simulink model "CRCL"  (R2020b)
settings: Solver=FixedStepDiscrete  StartTime=0.0  StopTime=inf  FixedStep=0.01  RelTol=1e-3  EnableMultiTasking=on
values from neighbouring files (symbols this model uses):
  calibrationDelayTime_s = 2.0    [CRCL_Dictionary.sldd]
  collisionAngleThreshold_deg = 40.0    [CRCL_Dictionary.sldd]
  collisionVarianceThreshold_g2 = 8.0    [CRCL_Dictionary.sldd]
  cpMaxAbortTime_s = 30.0    [CRCL_Dictionary.sldd]
  cpMaxTipOverAngle_deg = 35.0    [CRCL_Dictionary.sldd]
  cpMinEstDistance_m = 50.0    [CRCL_Dictionary.sldd]
  cpMinEstDistanceGnssBased_m = 200.0    [CRCL_Dictionary.sldd]
  cpMinRiddenTime_s = 15.0    [CRCL_Dictionary.sldd]
  cpMinSpeedRiding_kmh = 10.0    [CRCL_Dictionary.sldd]
  cpNumCrankRevolutionThreshold = 5.0    [CRCL_Dictionary.sldd]
  cpSpeedCond2PositiveSpeedChangeTime_s = 5.0    [CRCL_Dictionary.sldd]
  cpSpeedDerivativeThreshold_kmhs = 0.005    [CRCL_Dictionary.sldd]
  cpTimeOutSpeedCond2_s = 15.0    [CRCL_Dictionary.sldd]
  groundHitEnergyThresholdStanding_g2s2 = 0.02    [CRCL_Dictionary.sldd]
  groundHitTipOverAngleThreshold_deg = 40.0    [CRCL_Dictionary.sldd]
  longAccCompForEulerEstFlag = 0.0    [CRCL_Dictionary.sldd]
  minEnergyStrongHit_g2s2 = 0.1    [CRCL_Dictionary.sldd]
  noMotionAccVarianceThresholdSD_g2 = 0.001    [CRCL_Dictionary.sldd]
  ride1minSpeedSlow_kmh = 4.0    [CRCL_Dictionary.sldd]
  ride2minSpeed_kmh = 8.0    [CRCL_Dictionary.sldd]
  rroMaxSpeed_kmh = 5.0    [CRCL_Dictionary.sldd]
  rroMinGyrX_degs = 20.0    [CRCL_Dictionary.sldd]
  rroMonotonyThreshold_degs = -1.0    [CRCL_Dictionary.sldd]
  rroRollIntegrationAngleThreshold_degs = 20.0    [CRCL_Dictionary.sldd]
  rroUniContinuityThreshold_degs = 15.0    [CRCL_Dictionary.sldd]
  scaleFactorVarianceStrongHit = 2.0    [CRCL_Dictionary.sldd]
  sdoMaxAccVarFreeFall_g2 = 0.06    [CRCL_Dictionary.sldd]
  sdoMaxTipOverAngle_deg = 20.0    [CRCL_Dictionary.sldd]
  sdoMinAccVar_g2 = 8.0    [CRCL_Dictionary.sldd]
  sdoMinGyrXYNorm_degs = 720.0    [CRCL_Dictionary.sldd]
  sdoMinGyrXYNormFreeFall_degs = 100.0    [CRCL_Dictionary.sldd]
  sdoMinOrientationChange_deg = 120.0    [CRCL_Dictionary.sldd]
  sdoScaleFactorOrientationChange = 3.0    [CRCL_Dictionary.sldd]
  stepTime_s = 0.01    [CRCL_Dictionary.sldd]
  strongHitSafetyFactor = 2.5    [CRCL_Dictionary.sldd]
  tipOverAccZFiltTreshold_g = 0.7    [CRCL_Dictionary.sldd]
  tipOverAngleThreshold_deg = 50.0    [CRCL_Dictionary.sldd]
  tipOverMinAccZFiltNoseOver_g = 0.3    [CRCL_Dictionary.sldd]
  tipOverRollPitchRelationNoseOver = 1.5    [CRCL_Dictionary.sldd]
undefined symbols (not defined in the file or in its folder): magnitude
libraries: simulink x17
(part 5 of 8)

== stateflow chart CRCL/BikeCrashFusionProduct ==
  state CrashFusionAndDetection_SchneeV2_softHit2 [parallel] [commented out]
    state Init [commented out]
      en:
      CF_fire = int16(0);
      CF_checkTipOverTimeDelay = single(2);
      CF_possibleTo = single(0);
      HD_GroundHitFireIntern = int16(0);
      HD_CollisionHitFireIntern = int16(0);
    state RidingNotCalibratedTipOver [commented out]
      en:
      CF_fire = int16(1);
      CF_scenario = int16(70);
    state RidingNotCalibrated [commented out]
      en:
    state NoCrash [commented out]
      en:
      CF_scenario = int16(0);
      HD_CollisionHitFireIntern = int16(0);
      HD_GroundHitFireIntern = int16(0);
      du:
      CF_possibleTo = single(0);
    state waitUntilBikeIsUprightAgain [commented out]
    state wait2 [commented out]
      en:
      if CF_possibleTo == 0
      RD_fireIntern = RD_fire;
      end
      if HD_CollisionHitFire ==  1
      HD_CollisionHitFireIntern = int16(1);
      end
      CF_possibleTo = single(1);
    state HitDetected [commented out]
      %wait for possible Ground Hit and TipOver
      en:
      du:
      if HD_CollisionHitFire ==  3
      HD_CollisionHitFireIntern = int16(3);
      end
      if HD_GroundHitFire == 1
      HD_GroundHitFireIntern = int16(1);
      end
    state wait1 [commented out]
      en:
      if CF_possibleTo == 0
      RD_fireIntern = RD_fire;
      end
      if HD_CollisionHitFire ==  3
      HD_CollisionHitFireIntern = int16(3);
      elseif HD_CollisionHitFire ==  2
      HD_CollisionHitFireIntern = int16(2);
      elseif HD_CollisionHitFire ==  1
      HD_CollisionHitFireIntern = int16(1);
      end
      du:
      if HD_CollisionHitFire ==  2 && HD_CollisionHitFireIntern < 2
      HD_CollisionHitFireIntern = int16(2);
      end
      if HD_CollisionHitFire == 3 && HD_CollisionHitFireIntern < 3
      HD_CollisionHitFireIntern = int16(3);
      end
    state wait [commented out]
      du:
      if HD_GroundHitFire == 1
      HD_GroundHitFireIntern = int16(1);
      end
      ex:
      if HD_GroundHitFire == 1
      HD_GroundHitFireIntern = int16(1);
      end
      if HD_CollisionHitFire ==  3
      HD_CollisionHitFireIntern = int16(3);
      elseif HD_CollisionHitFire ==  2
      HD_CollisionHitFireIntern = int16(2);
      elseif HD_CollisionHitFire ==  1
      HD_CollisionHitFireIntern = int16(1);
      end
    note: ______________________________________________________________________________________________________________________________________________________________________________________________v Ride Feature Layer v
    note: ______________________________________________________________________________________________________________________________________________________________________________________________v CollisionHit Feature Layer v
    note: ______________________________________________________________________________________________________________________________________________________________________________________________v GroundHit Feature Layer v
    note: ____________________________________________________________________________________________________________________________________________________________________________________________________________v TipOver Feature Layer v
    note: ____________________________________________________________________________________________________________________________________________________________________________________________________________v StrongHit Feature Layer v
    note: _________________________________________________________________________________________________________________________________________________________________________________________________________________v Classifcation Layer v
    state Crash [commented out]
      en:
      if ~(CF_scenario == 70)
      CF_fire = int16(1);
      end
    (default) -> CrashFusionAndDetection_SchneeV2_softHit2.Init [commented out]
    CrashFusionAndDetection_SchneeV2_softHit2.RidingNotCalibratedTipOver -> CrashFusionAndDetection_SchneeV2_softHit2.Init [commented out] : [after(5,sec) && TO_fire == 0]
        | {
        | CF_fire = int16(0);
        | CF_scenario = int16(0);
        | }
    CrashFusionAndDetection_SchneeV2_softHit2.RidingNotCalibrated -> CrashFusionAndDetection_SchneeV2_softHit2.Init [commented out] : [RD_fire < 2]
    CrashFusionAndDetection_SchneeV2_softHit2.RidingNotCalibrated -> CrashFusionAndDetection_SchneeV2_softHit2.RidingNotCalibratedTipOver [commented out] : [TO_fire == 3]
    CrashFusionAndDetection_SchneeV2_softHit2.Init -> CrashFusionAndDetection_SchneeV2_softHit2.RidingNotCalibrated [commented out] : [CF_systemConfig == 2 && RD_fire >= 2 && TO_fire ~= 3]
    CrashFusionAndDetection_SchneeV2_softHit2.RidingNotCalibrated -> CrashFusionAndDetection_SchneeV2_softHit2.NoCrash [commented out] : [HD_secondCalibrationDone == 1]
    CrashFusionAndDetection_SchneeV2_softHit2.Init -> CrashFusionAndDetection_SchneeV2_softHit2.NoCrash [commented out] : [HD_secondCalibrationDone ==1]
    CrashFusionAndDetection_SchneeV2_softHit2.waitUntilBikeIsUprightAgain -> CrashFusionAndDetection_SchneeV2_softHit2.NoCrash [commented out] : [TO_fire == 0]
    CrashFusionAndDetection_SchneeV2_softHit2.Crash -> CrashFusionAndDetection_SchneeV2_softHit2.waitUntilBikeIsUprightAgain [commented out] : %[after(5,sec) && TO_fire == 0 && ~(CF_hubConnection == 0 && ...
        |  %CF_systemConfig == 2 && CF_cobiHubSetup ~= 1) && CF_sdoFire == 0]
        | [after(7,sec)]
        | {
        | CF_fire = int16(0);
        | CF_possibleTo = single(0);
        | }
    (junction 644) -> CrashFusionAndDetection_SchneeV2_softHit2.NoCrash [commented out]
    CrashFusionAndDetection_SchneeV2_softHit2.NoCrash -> CrashFusionAndDetection_SchneeV2_softHit2.HitDetected [commented out] : [HD_CollisionHitFire >= 2]
        | {
        | HD_CollisionHitFireIntern = int16(2);
        | RD_fireIntern = RD_fire; % take RD_flag during Collision
        | % backWheel might start rotating after Crash
        | % -> wrong crash classification
        | }
    CrashFusionAndDetection_SchneeV2_softHit2.NoCrash -> (junction 611) [commented out] : [CF_hubConnection == 1 && ...
        |  CF_sdoFire == 1 && ...
        |  CF_systemConfig == 2]
        | {
        | RD_fireIntern = RD_fire;
        | }
    CrashFusionAndDetection_SchneeV2_softHit2.NoCrash -> CrashFusionAndDetection_SchneeV2_softHit2.wait1 [commented out] : [HD_GroundHitFire ==1]
        | {
        | HD_GroundHitFireIntern = int16(1);
        | }
    CrashFusionAndDetection_SchneeV2_softHit2.wait1 -> CrashFusionAndDetection_SchneeV2_softHit2.NoCrash [commented out] : [after(CF_checkTipOverTimeDelay,sec)]
    CrashFusionAndDetection_SchneeV2_softHit2.wait -> CrashFusionAndDetection_SchneeV2_softHit2.NoCrash [commented out] : [after(CF_checkTipOverTimeDelay/2+0.1,sec) && ...
        | TO_fire == 0]
    CrashFusionAndDetection_SchneeV2_softHit2.wait2 -> CrashFusionAndDetection_SchneeV2_softHit2.NoCrash [commented out] : [after(CF_checkTipOverTimeDelay/2+0.1,sec) || ...
        | TO_fire == 0]
    CrashFusionAndDetection_SchneeV2_softHit2.NoCrash -> CrashFusionAndDetection_SchneeV2_softHit2.wait2 [commented out] : [TO_fire >= 0.5]
    CrashFusionAndDetection_SchneeV2_softHit2.wait2 -> CrashFusionAndDetection_SchneeV2_softHit2.wait [commented out] : [TO_fire >= 1]
        | {
        | TO_fireIntern = TO_fire;
        | }
    CrashFusionAndDetection_SchneeV2_softHit2.wait2 -> (junction 612) [commented out] : %cobi hub lost
        | [CF_hubConnection == 0 && ...
        | (HD_GroundHitFire == 1 || HD_CollisionHitFire >= 2) && ...
        | CF_systemConfig == 2 && CF_cobiHubSetup ~= 1]
        | {
        | HD_GroundHitFireIntern = HD_GroundHitFire;
        | HD_CollisionHitFireIntern = HD_CollisionHitFire;
        | }
    CrashFusionAndDetection_SchneeV2_softHit2.HitDetected -> (junction 611) [commented out] : [HD_CollisionHitFire == 0 || ...
        | (after(CF_checkTipOverTimeDelay,sec) && TO_fire >= 1) ||...
        | (CF_hubConnection == 0 && CF_systemConfig == 2 && ...
        | CF_cobiHubSetup ~= 1)]
        | {
        | TO_fireIntern = TO_fire;
        | }
    CrashFusionAndDetection_SchneeV2_softHit2.wait1 -> (junction 612) [commented out] : [TO_fire >= 1 ||...
        | (CF_hubConnection == 0 && CF_systemConfig == 2 && ...
        | CF_cobiHubSetup ~= 1)]
        | {
        | TO_fireIntern = TO_fire;
        | }
    CrashFusionAndDetection_SchneeV2_softHit2.wait -> (junction 612) [commented out] : [after(CF_checkTipOverTimeDelay/2,sec)]
    (junction 611) -> (junction 773) [commented out] : [CF_hubConnection == 1 && CF_sdoFire == 1 && CF_systemConfig == 2]
    (junction 612) -> (junction 773) [commented out] : [CF_hubConnection == 1 && CF_sdoFire == 1 && CF_systemConfig == 2]
    (junction 611) -> (junction 765) [commented out] : [CF_hubConnection == 0 && CF_systemConfig == 2 && CF_cobiHubSetup ~= 1 &&...
        | (HD_GroundHitFireIntern == 1 || HD_CollisionHitFireIntern >= 2 || RD_fireIntern >= 2)]
    (junction 612) -> (junction 765) [commented out] : [CF_hubConnection == 0 && CF_systemConfig == 2 && CF_cobiHubSetup ~= 1 &&...
        | (HD_GroundHitFireIntern == 1 || HD_CollisionHitFireIntern >= 2 || RD_fireIntern >= 2)]
    (junction 612) -> (junction 613) [commented out] : [RD_fireIntern >= 2]
    (junction 611) -> (junction 614) [commented out]
    (junction 611) -> (junction 613) [commented out] : [RD_fireIntern >= 1]
    (junction 612) -> (junction 614) [commented out]
    (junction 773) -> (junction 796) [commented out] : % smartphoneDropOut: class 82 or 83
        | {
        | CF_scenario = int16(82);
        | }
    (junction 765) -> (junction 788) [commented out] : % cobi hub lost: class 80 or 81
        | {
        | CF_scenario = int16(80);
        | }
    (junction 614) -> (junction 617) [commented out] : [HD_CollisionHitFireIntern >= 2]
    (junction 614) -> (junction 618) [commented out]
    (junction 613) -> (junction 620) [commented out] : [HD_CollisionHitFireIntern >= 2]
    (junction 613) -> (junction 622) [commented out]
    (junction 618) -> (junction 626) [commented out] : % this path is not reachable?
    (junction 617) -> (junction 623) [commented out] : [HD_GroundHitFireIntern == 1 ...
        | && TO_fireIntern >= 1]
    (junction 618) -> (junction 625) [commented out] : [HD_GroundHitFireIntern == 1 ...
        | && TO_fireIntern >= 1]
    (junction 617) -> (junction 624) [commented out]
    (junction 625) -> (junction 623) [commented out] : [HD_CollisionHitFireIntern >= 1 &&...
        | RD_fireIntern == 0]
    (junction 620) -> (junction 627) [commented out] : [TO_fireIntern == 1]
    (junction 625) -> (junction 750) [commented out] : [RRO_fire == 1 && ...
        | RD_fireIntern == 0]
    (junction 624) -> (junction 623) [commented out] : [TO_fireIntern >= 1]
    (junction 624) -> (junction 634) [commented out]
    (junction 626) -> (junction 636) [commented out]
    (junction 620) -> (junction 628) [commented out] : [TO_fireIntern == 2]
    (junction 622) -> (junction 633) [commented out]
    (junction 622) -> (junction 631) [commented out] : [TO_fireIntern == 1]
    (junction 620) -> (junction 629) [commented out]
    (junction 625) -> (junction 777) [commented out] : %crash scenario 3X
    (junction 622) -> (junction 632) [commented out] : [TO_fireIntern == 2]
    (junction 623) -> (junction 637) [commented out]
    (junction 626) -> (junction 635) [commented out] : [TO_fireIntern >= 1]
    (junction 631) -> (junction 627) [commented out] : [HD_SoftCollisionFire == 1]
    (junction 629) -> (junction 639) [commented out]
    (junction 637) -> (junction 643) [commented out] : [TO_fireIntern == 2 || TO_NoseOverFireIntern == 1]
    (junction 634) -> (junction 641) [commented out]
    (junction 634) -> (junction 640) [commented out] : [HD_CollisionHitFireIntern >= 3]
        | %&& HD_CollisionFrontRearLat == 1]
    (junction 637) -> (junction 642) [commented out]
    (junction 627) -> (junction 815) [commented out]
    (junction 628) -> (junction 820) [commented out]
    (junction 629) -> (junction 737) [commented out] : [HD_StrongCollisionHitFireIntern == 1 && ...
        | HD_CollisionFrontRearLat == 1]
    (junction 627) -> (junction 816) [commented out] : [HD_CollisionHitFireIntern >= 3]
    (junction 629) -> (junction 638) [commented out] : [HD_CollisionHitFireIntern >= 3 ]
        | % && ... HD_CollisionFrontRearLat == 1]
    (junction 628) -> (junction 821) [commented out] : [HD_CollisionHitFireIntern >= 3]
    (junction 636) -> (junction 649) [commented out] : %no crash
    (junction 635) -> (junction 648) [commented out] : %crash scenario 9
        | %no crash!!!
    (junction 631) -> CrashFusionAndDetection_SchneeV2_softHit2.Crash [commented out] : %crash scenario 20
        | {
        | CF_scenario = int16(20);
        | ;}
    (junction 632) -> CrashFusionAndDetection_SchneeV2_softHit2.Crash [commented out] : %crash scenario 22
        | {
        | CF_scenario = int16(22);
        | }
    (junction 633) -> (junction 646) [commented out] : %no crash!
    (junction 750) -> CrashFusionAndDetection_SchneeV2_softHit2.Crash [commented out] : %crash scenario 70
        | {
        | CF_scenario = int16(70);
        | }
    (junction 639) -> (junction 642) [commented out]
    (junction 777) -> CrashFusionAndDetection_SchneeV2_softHit2.Crash [commented out] : [RD_fireIntern == 0 && ...
        | TO_fireIntern >= 1]
        | {
        | CF_scenario = int16(33);
        | }
    (junction 777) -> CrashFusionAndDetection_SchneeV2_softHit2.Crash [commented out] : {
        | CF_scenario = int16(30);
        | }
    (junction 642) -> (junction 808) [commented out]
    (junction 642) -> (junction 807) [commented out] : [HD_CollisionHitFireIntern == 3]
    (junction 815) -> CrashFusionAndDetection_SchneeV2_softHit2.Crash [commented out] : %crash scenario 10
        | {
        | CF_scenario = int16(10);
        | }
    (junction 816) -> CrashFusionAndDetection_SchneeV2_softHit2.Crash [commented out] : %crash scenario 15
        | {
        | CF_scenario = int16(15);
        | }
    (junction 820) -> CrashFusionAndDetection_SchneeV2_softHit2.Crash [commented out] : %crash scenario 12
        | {
        | CF_scenario = int16(12);
        | }
    (junction 821) -> CrashFusionAndDetection_SchneeV2_softHit2.Crash [commented out] : %crash scenario 16
        | {
        | CF_scenario = int16(16);
        | }
    (junction 638) -> CrashFusionAndDetection_SchneeV2_softHit2.Crash [commented out] : %crash scenario 11
        | {
        | CF_scenario = int16(11);
        | }
    (junction 737) -> CrashFusionAndDetection_SchneeV2_softHit2.Crash [commented out] : %crash scenario 2
        | {
        | CF_scenario = int16(25);
        | }
    (junction 639) -> (junction 645) [commented out] : %no crash
    (junction 642) -> (junction 806) [commented out] : [HD_CollisionHitFireIntern == 2]
    (junction 643) -> CrashFusionAndDetection_SchneeV2_softHit2.Crash [commented out] : %crash scenario 42
        | {
        | CF_scenario = int16(42);
        | }
    (junction 640) -> CrashFusionAndDetection_SchneeV2_softHit2.Crash [commented out] : %crash scenario 41
        | {
        | CF_scenario = int16(41);
        | }
    (junction 641) -> (junction 647) [commented out] : %no crash
    (junction 777) -> CrashFusionAndDetection_SchneeV2_softHit2.Crash [commented out] : [RD_fireIntern == 1 && ...
        |  TO_fireIntern == 2]
        | {
        | CF_scenario = int16(32);
        | }
    (junction 645) -> (junction 644) [commented out]
    (junction 646) -> (junction 645) [commented out]
    (junction 647) -> (junction 646) [commented out]
    (junction 648) -> (junction 647) [commented out]
    (junction 649) -> (junction 648) [commented out]
    (junction 788) -> (junction 792) [commented out]
    (junction 796) -> (junction 798) [commented out]
    (junction 788) -> (junction 791) [commented out] : [RD_fireIntern >= 1]
    (junction 796) -> (junction 800) [commented out] : [RD_fireIntern >= 1]
    (junction 808) -> CrashFusionAndDetection_SchneeV2_softHit2.Crash [commented out] : %crash scenario 40
        | {
        | CF_scenario = int16(40);
        | }
    (junction 806) -> CrashFusionAndDetection_SchneeV2_softHit2.Crash [commented out] : %crash scenario 44
        | {
        | CF_scenario = int16(44);
        | }
    (junction 807) -> CrashFusionAndDetection_SchneeV2_softHit2.Crash [commented out] : %crash scenario 45
        | {
        | CF_scenario = int16(45);
        | }
    (junction 791) -> CrashFusionAndDetection_SchneeV2_softHit2.Crash [commented out] : {
        | CF_scenario = int16(81);
        | }
    (junction 792) -> CrashFusionAndDetection_SchneeV2_softHit2.Crash [commented out] : {
        | CF_scenario = int16(80);
        | }
    (junction 800) -> CrashFusionAndDetection_SchneeV2_softHit2.Crash [commented out] : {
        | CF_scenario = int16(83);
        | }
    (junction 798) -> CrashFusionAndDetection_SchneeV2_softHit2.Crash [commented out] : {
        | CF_scenario = int16(82);
        | }
    CrashFusionAndDetection_SchneeV2_softHit2.Crash -> CrashFusionAndDetection_SchneeV2_softHit2.Crash [commented out] : %smartphoneDropoutdetected after first crash classification
        | [~any(CF_scenario == [82 81 80]) && ...
        | CF_hubConnection == 1 && ...
        | CF_sdoFire == 1 && ...
        | CF_systemConfig == 2 && ...
        | RD_fireIntern == 0]
        | {
        | CF_scenario = int16(82);
        | }
    CrashFusionAndDetection_SchneeV2_softHit2.Crash -> CrashFusionAndDetection_SchneeV2_softHit2.Crash [commented out] : %smartphoneDropoutdetected after first crash classification
        | [~any(CF_scenario == [83 81 80]) && ...
        | CF_hubConnection == 1 && ...
        | CF_sdoFire == 1 && ...
        | CF_systemConfig == 2 && ...
        | RD_fireIntern >= 1]
        | {
        | CF_scenario = int16(83);
        | }
    CrashFusionAndDetection_SchneeV2_softHit2.Crash -> CrashFusionAndDetection_SchneeV2_softHit2.Crash [commented out] : %cobiHubLost after first crash classification
        | [CF_scenario ~= 81 && ...
        | RD_fireIntern >= 1 && CF_hubConnection == 0 && CF_cobiHubSetup ~= 1  && ...
        | CF_systemConfig == 2 && ...
        | (HD_GroundHitFireIntern == 1 || HD_CollisionHitFireIntern >= 2)]
        | {
        | CF_scenario = int16(81);
        | }
    CrashFusionAndDetection_SchneeV2_softHit2.Crash -> CrashFusionAndDetection_SchneeV2_softHit2.Crash [commented out] : %cobiHubLost after first crash classification
        | [CF_scenario ~= 80 && ...
        | RD_fireIntern == 0 && CF_hubConnection == 0 && CF_cobiHubSetup ~= 1 && ...
        | CF_systemConfig == 2 && ...
        | (HD_GroundHitFireIntern == 1 || HD_CollisionHitFireIntern >= 2)]
        | {
        | CF_scenario = int16(80);
        | }
  state CrashFusionAndDetection_SchneeV2_softHit3 [parallel]
    settings: executionOrder=1
    state Init
      en:
      CF_fire = int16(0);
      CF_checkTipOverTimeDelay = single(2);
      CF_possibleTo = logical(0);
      HD_GroundHitFireIntern = int16(0);
      HD_CollisionHitFireIntern = int16(0);
    state RidingNotCalibratedTipOver [commented out]
      en:
      CF_fire = int16(1);
      CF_scenario = int16(70);
    state RidingNotCalibrated [commented out]
      en:
    state NoCrash
      en:
      CF_scenario = int16(0);
      HD_CollisionHitFireIntern = int16(0);
      HD_GroundHitFireIntern = int16(0);
      du:
      CF_possibleTo = logical(0);
    state waitUntilBikeIsUprightAgain
    note: Enter here when a collision was seen and bike is still upright
    state wait2
      en:
      if CF_possibleTo == 0
      RD_fireIntern = RD_fire;
      end
      if HD_CollisionHitFire ==  1
      HD_CollisionHitFireIntern = int16(1);
      end
      CF_possibleTo = logical(1);
    state HitDetected
      %wait for possible Ground Hit and TipOver
      en:
      du:
      if HD_CollisionHitFire ==  3
      HD_CollisionHitFireIntern = int16(3);
      end
      if HD_GroundHitFire == 1
      HD_GroundHitFireIntern = int16(1);
      end
    state wait1
      en:
      if CF_possibleTo == 0
      RD_fireIntern = RD_fire;
      end
      if HD_CollisionHitFire ==  3 && ...
      ~(CF_systemConfig == 2 && CF_bikeStillUpright == 0)
      HD_CollisionHitFireIntern = int16(3);
      elseif HD_CollisionHitFire ==  2 && ...
      ~(CF_systemConfig == 2 && CF_bikeStillUpright == 0)
      HD_CollisionHitFireIntern = int16(2);
      elseif HD_CollisionHitFire ==  1 && ...
      ~(CF_systemConfig == 2 && CF_bikeStillUpright == 0)
      HD_CollisionHitFireIntern = int16(1);
      end
      du:
      if HD_CollisionHitFire ==  2 && HD_CollisionHitFireIntern < 2 && ...
      ~(CF_systemConfig == 2 && CF_bikeStillUpright == 0)
      HD_CollisionHitFireIntern = int16(2);
      end
      if HD_CollisionHitFire == 3 && HD_CollisionHitFireIntern < 3 && ...
      ~(CF_systemConfig == 2 && CF_bikeStillUpright == 0)
      HD_CollisionHitFireIntern = int16(3);
      end
    state wait
      du:
      if HD_GroundHitFire == 1
      HD_GroundHitFireIntern = int16(1);
      end
      ex:
      if HD_GroundHitFire == 1
      HD_GroundHitFireIntern = int16(1);
      end
      if HD_CollisionHitFire ==  3
      HD_CollisionHitFireIntern = int16(3);
      elseif HD_CollisionHitFire ==  2
      HD_CollisionHitFireIntern = int16(2);
      elseif HD_CollisionHitFire ==  1
      HD_CollisionHitFireIntern = int16(1);
      end
    note: ______________________________________________________________________________________________________________________________________________________________________________________________v Ride Feature Layer v
    note: ______________________________________________________________________________________________________________________________________________________________________________________________v CollisionHit Feature Layer v
    note: ______________________________________________________________________________________________________________________________________________________________________________________________v GroundHit Feature Layer v
    note: ____________________________________________________________________________________________________________________________________________________________________________________________________________v TipOver Feature Layer v
    note: ____________________________________________________________________________________________________________________________________________________________________________________________________________v StrongHit Feature Layer v
    note: _________________________________________________________________________________________________________________________________________________________________________________________________________________v Classifcation Layer v
    state Crash
      en:
      if ~(CF_scenario == 70)
      CF_fire = int16(1);
      end
    (default) -> CrashFusionAndDetection_SchneeV2_softHit3.Init
    CrashFusionAndDetection_SchneeV2_softHit3.RidingNotCalibratedTipOver -> CrashFusionAndDetection_SchneeV2_softHit3.Init [commented out] : [after(5,sec) && TO_fire == 0]
        | {
        | CF_fire = int16(0);
        | CF_scenario = int16(0);
        | }
    CrashFusionAndDetection_SchneeV2_softHit3.RidingNotCalibrated -> CrashFusionAndDetection_SchneeV2_softHit3.Init [commented out] : [RD_fire < 2]
    CrashFusionAndDetection_SchneeV2_softHit3.RidingNotCalibrated -> CrashFusionAndDetection_SchneeV2_softHit3.RidingNotCalibratedTipOver [commented out] : [TO_fire == 3]
    CrashFusionAndDetection_SchneeV2_softHit3.Init -> CrashFusionAndDetection_SchneeV2_softHit3.RidingNotCalibrated [commented out] : [CF_systemConfig == 2 && RD_fire >= 2 && TO_fire ~= 3]
    CrashFusionAndDetection_SchneeV2_softHit3.RidingNotCalibrated -> CrashFusionAndDetection_SchneeV2_softHit3.NoCrash [commented out] : [HD_secondCalibrationDone == 1]
    CrashFusionAndDetection_SchneeV2_softHit3.Init -> CrashFusionAndDetection_SchneeV2_softHit3.NoCrash : [HD_secondCalibrationDone ==1]
    CrashFusionAndDetection_SchneeV2_softHit3.waitUntilBikeIsUprightAgain -> CrashFusionAndDetection_SchneeV2_softHit3.NoCrash : [TO_fire == 0 && CF_sdoFire == 0] % && ...
        | %(CF_hubConnection == 1 || CF_systemConfig ~= 2 || CF_cobiHubSetup == 1)]
        | % this second line of conditions, waits until the HubConnection is back online,
        | % before another crash can be detected (only for cobi ebike case)
    CrashFusionAndDetection_SchneeV2_softHit3.Crash -> CrashFusionAndDetection_SchneeV2_softHit3.waitUntilBikeIsUprightAgain [order 3] : %[after(5,sec) && TO_fire == 0 && ~(CF_hubConnection == 0 && ...
        |  %CF_systemConfig == 2 && CF_cobiHubSetup ~= 1) && CF_sdoFire == 0]
        | [after(7,sec)]
        | {
        | CF_fire = int16(0);
        | CF_possibleTo = logical(0);
        | CF_scenario = int16(0);
        | }
    (junction 870) -> CrashFusionAndDetection_SchneeV2_softHit3.NoCrash
    CrashFusionAndDetection_SchneeV2_softHit3.NoCrash -> CrashFusionAndDetection_SchneeV2_softHit3.HitDetected [order 2] : [HD_CollisionHitFire >= 2 && ...
        | ~(CF_systemConfig == 2 && CF_bikeStillUpright == 0)]
        | {
        | HD_CollisionHitFireIntern = int16(2);
        | RD_fireIntern = RD_fire; % take RD_flag during Collision
        | % backWheel might start rotating after Crash
        | % -> wrong crash classification
        | }
    CrashFusionAndDetection_SchneeV2_softHit3.NoCrash -> (junction 833) [order 4] : [CF_hubConnection == 1 && ...
        |  CF_sdoFire == 2 && ...
        |  CF_systemConfig == 2]
        | {
        | RD_fireIntern = RD_fire;
        | TO_fireIntern = TO_fire;
        | }
    CrashFusionAndDetection_SchneeV2_softHit3.NoCrash -> CrashFusionAndDetection_SchneeV2_softHit3.wait1 [order 1] : [HD_GroundHitFire ==1]
        | {
        | HD_GroundHitFireIntern = int16(1);
        | }
    CrashFusionAndDetection_SchneeV2_softHit3.wait1 -> CrashFusionAndDetection_SchneeV2_softHit3.NoCrash [order 2] : [after(CF_checkTipOverTimeDelay,sec)]
    CrashFusionAndDetection_SchneeV2_softHit3.wait -> CrashFusionAndDetection_SchneeV2_softHit3.NoCrash [order 2] : [after(CF_checkTipOverTimeDelay/2+0.1,sec) && ...
        | TO_fire == 0]
    CrashFusionAndDetection_SchneeV2_softHit3.wait2 -> CrashFusionAndDetection_SchneeV2_softHit3.NoCrash [order 1] : [after(CF_checkTipOverTimeDelay/2+0.1,sec) || ...
        | TO_fire == 0]
    CrashFusionAndDetection_SchneeV2_softHit3.NoCrash -> CrashFusionAndDetection_SchneeV2_softHit3.wait2 [order 3] : [TO_fire >= 1]
    CrashFusionAndDetection_SchneeV2_softHit3.wait2 -> CrashFusionAndDetection_SchneeV2_softHit3.wait [order 2] : [TO_fire >= 2]
        | {
        | TO_fireIntern = TO_fire;
        | }
    CrashFusionAndDetection_SchneeV2_softHit3.wait2 -> (junction 834) [order 3] : %cobi hub lost
        | [CF_hubConnection == 0 && ...
        | (HD_GroundHitFire == 1 || HD_CollisionHitFire >= 2) && ...
        | CF_systemConfig == 2 && CF_cobiHubSetup ~= 1]
        | {
        | HD_GroundHitFireIntern = HD_GroundHitFire;
        | HD_CollisionHitFireIntern = HD_CollisionHitFire;
        | TO_fireIntern = TO_fire;
        | }
    CrashFusionAndDetection_SchneeV2_softHit3.HitDetected -> (junction 833) : [HD_CollisionHitFire == 0 || ...
        | (after(CF_checkTipOverTimeDelay,sec) && TO_fire >= 2) ||...
        | (CF_hubConnection == 0 && CF_systemConfig == 2 && ...
        | CF_cobiHubSetup ~= 1)]
        | {
        | TO_fireIntern = TO_fire;
        | }
    CrashFusionAndDetection_SchneeV2_softHit3.wait1 -> (junction 834) [order 1] : [TO_fire >= 2 ||...
        | (CF_hubConnection == 0 && CF_systemConfig == 2 && ...
        | CF_cobiHubSetup ~= 1)]
        | {
        | TO_fireIntern = TO_fire;
        | }
    CrashFusionAndDetection_SchneeV2_softHit3.wait -> (junction 834) [order 1] : [after(CF_checkTipOverTimeDelay/2,sec)]
    (junction 833) -> (junction 836) [order 2] : [CF_hubConnection == 0 && CF_systemConfig == 2 && CF_cobiHubSetup ~= 1 &&...
        | (HD_GroundHitFireIntern == 1 || HD_CollisionHitFireIntern >= 2 || RD_fireIntern >= 2)]
    (junction 834) -> (junction 836) [order 2] : [CF_hubConnection == 0 && CF_systemConfig == 2 && CF_cobiHubSetup ~= 1 &&...
        | (HD_GroundHitFireIntern == 1 || HD_CollisionHitFireIntern >= 2 || RD_fireIntern >= 2)]
    (junction 833) -> (junction 835) [order 1] : [CF_hubConnection == 1 && CF_sdoFire == 2 && CF_systemConfig == 2]
    (junction 834) -> (junction 835) [order 1] : [CF_hubConnection == 1 && CF_sdoFire == 2 && CF_systemConfig == 2]
    (junction 833) -> (junction 838) [order 4]
    (junction 834) -> (junction 837) [order 3] : [RD_fireIntern >= 2]
    (junction 833) -> (junction 837) [order 3] : [RD_fireIntern >= 1]
    (junction 834) -> (junction 838) [order 4]
    CrashFusionAndDetection_SchneeV2_softHit3.Crash -> (junction 835) [order 1] : %smartphoneDropoutdetected after first crash classification
        | [CF_scenario < 80 && ...
        | (CF_hubConnection == 1 || ...
        | CF_cobiHubSetup == 1) && ... %hubCon not necessary for bioBike cases
        | CF_sdoFire == 2 && ...
        | CF_systemConfig == 2]
    CrashFusionAndDetection_SchneeV2_softHit3.Crash -> (junction 836) [order 2] : %smartphoneDropoutdetected after first crash classification
        | [CF_scenario < 90 && ...
        | CF_hubConnection == 0 && ...
        | CF_cobiHubSetup ~= 1 && ... %hubConnectionLost cases not for bioBike!
        | CF_systemConfig == 2]
    (junction 835) -> (junction 1017) : % smartphoneDropOut,
        | % but still hub connection
    (junction 836) -> (junction 876) : % cobi hub lost:
    (junction 1017) -> (junction 1018) [order 2]
    (junction 876) -> (junction 1047) [order 2]
    (junction 1017) -> (junction 1020) [order 1] : [RD_fireIntern >= 1]
    (junction 876) -> (junction 1028) [order 1] : [RD_fireIntern >= 1]
    (junction 1020) -> (junction 1022) [order 2]
    (junction 1028) -> (junction 1037) [order 2]
    (junction 1020) -> (junction 1013) [order 1] : [HD_CollisionHitFireIntern >=2]
    (junction 1028) -> (junction 1029) [order 1] : [HD_CollisionHitFireIntern >=2]
    (junction 1018) -> (junction 883) [order 2]
    (junction 1047) -> (junction 1042) [order 2]
    (junction 1018) -> (junction 884) [order 1] : [HD_CollisionHitFireIntern >=2]
    (junction 1047) -> (junction 1043) [order 1] : [HD_CollisionHitFireIntern >=2]
    (junction 838) -> (junction 839) [order 1] : [HD_CollisionHitFireIntern >= 2]
    (junction 838) -> (junction 840) [order 2]
    (junction 837) -> (junction 841) [order 1] : [HD_CollisionHitFireIntern >= 2]
    (junction 837) -> (junction 842) [order 2]
    (junction 840) -> (junction 846) [order 2] : % this path is not reachable?
    (junction 839) -> (junction 843) [order 1] : [HD_GroundHitFireIntern == 1 ...
        | && TO_fireIntern >= 2]
    (junction 840) -> (junction 845) [order 1] : [HD_GroundHitFireIntern == 1 ...
        | && TO_fireIntern >= 2]
    (junction 839) -> (junction 844) [order 2]
    (junction 845) -> (junction 843) [order 1] : [HD_CollisionHitFireIntern >= 1 &&...
        | RD_fireIntern == 0]
    (junction 841) -> (junction 847) [order 1] : [TO_fireIntern == 2]
    (junction 845) -> (junction 855) [order 2] : [RRO_fire == 1 && ...
        | RD_fireIntern == 0]
    (junction 844) -> (junction 843) [order 1] : [TO_fireIntern >= 2]
    (junction 844) -> (junction 854) [order 2]
    (junction 846) -> (junction 857) [order 2]
    (junction 841) -> (junction 848) [order 2] : [TO_fireIntern == 3]
    (junction 842) -> (junction 852) [order 3]
    (junction 842) -> (junction 850) [order 1] : [TO_fireIntern == 2]
    (junction 841) -> (junction 849) [order 3]
    (junction 845) -> (junction 869) [order 3] : %crash scenario 3X
    (junction 842) -> (junction 851) [order 2] : [TO_fireIntern == 3]
    (junction 843) -> (junction 853)
    (junction 846) -> (junction 856) [order 1] : [TO_fireIntern >= 2]
    (junction 1022) -> (junction 1051) [order 2]
    (junction 1037) -> (junction 1056) [order 2]
    (junction 1022) -> (junction 1015) [order 1] : [TO_fireIntern >= 2 && ...
        | CF_cobiHubSetup == 2]
    (junction 1037) -> (junction 1031) [order 1] : [TO_fireIntern >= 2 && ...
        | CF_cobiHubSetup == 2]
    (junction 850) -> (junction 847) [commented out] : [HD_SoftCollisionFire == 1]
    (junction 849) -> (junction 864) [order 2]
    (junction 853) -> (junction 866) [commented out] : [TO_fireIntern == 2 || TO_NoseOverFireIntern == 1]
    (junction 854) -> (junction 868) [order 2]
    (junction 854) -> (junction 867) [order 1] : [HD_CollisionHitFireIntern >= 3]
        | %&& HD_CollisionFrontRearLat == 1]
    (junction 853) -> (junction 865)
    (junction 847) -> (junction 858) [order 2]
    (junction 848) -> (junction 860) [order 2]
    (junction 849) -> (junction 863) [commented out] : [HD_StrongCollisionHitFireIntern == 1 && ...
        | HD_CollisionFrontRearLat == 1]
    (junction 847) -> (junction 859) [order 1] : [HD_CollisionHitFireIntern >= 3]
    (junction 849) -> (junction 862) [order 1] : [HD_CollisionHitFireIntern >= 3 ]
        | % && ... HD_CollisionFrontRearLat == 1]
    (junction 848) -> (junction 861) [order 1] : [HD_CollisionHitFireIntern >= 3]
    (junction 857) -> (junction 875) : %no crash
    (junction 850) -> CrashFusionAndDetection_SchneeV2_softHit3.Crash : %crash scenario 20
        | {
        | CF_scenario = int16(20);
        | ;}
    (junction 851) -> CrashFusionAndDetection_SchneeV2_softHit3.Crash : %crash scenario 22
        | {
        | CF_scenario = int16(22);
        | }
    (junction 852) -> (junction 872) : %no crash!
    (junction 855) -> CrashFusionAndDetection_SchneeV2_softHit3.Crash : %crash scenario 70
        | {
        | CF_scenario = int16(70);
        | }
    (junction 856) -> (junction 874) : %crash scenario 9
        | %no crash!!!
    (junction 864) -> (junction 865) [commented out]
    (junction 869) -> CrashFusionAndDetection_SchneeV2_softHit3.Crash [order 1] : [RD_fireIntern == 0 && ...
        | TO_fireIntern >= 2]
        | {
        | CF_scenario = int16(33);
        | }
    (junction 869) -> CrashFusionAndDetection_SchneeV2_softHit3.Crash [order 3] : {
        | CF_scenario = int16(30);
        | }
    (junction 865) -> (junction 878) [order 3]
    (junction 865) -> (junction 880) [order 1] : [HD_CollisionHitFireIntern == 3]
    (junction 1056) -> (junction 1034) [order 2]
    (junction 1051) -> (junction 1011) [order 2]
    (junction 1051) -> (junction 1052) [order 1] : [CF_cobiHubSetup == 2]
    (junction 1056) -> (junction 1059) [order 1] : [CF_cobiHubSetup == 2]
    (junction 858) -> CrashFusionAndDetection_SchneeV2_softHit3.Crash : %crash scenario 10
        | {
        | CF_scenario = int16(10);
        | }
    (junction 859) -> CrashFusionAndDetection_SchneeV2_softHit3.Crash : %crash scenario 15
        | {
        | CF_scenario = int16(15);
        | }
    (junction 860) -> CrashFusionAndDetection_SchneeV2_softHit3.Crash : %crash scenario 12
        | {
        | CF_scenario = int16(12);
        | }
    (junction 861) -> CrashFusionAndDetection_SchneeV2_softHit3.Crash : %crash scenario 16
        | {
        | CF_scenario = int16(16);
        | }
    (junction 862) -> CrashFusionAndDetection_SchneeV2_softHit3.Crash : %crash scenario 11
        | {
        | CF_scenario = int16(11);
        | }
    (junction 863) -> CrashFusionAndDetection_SchneeV2_softHit3.Crash [commented out] : %crash scenario 2
        | {
        | CF_scenario = int16(25);
        | }
    (junction 864) -> (junction 871) : %no crash
    (junction 865) -> (junction 879) [order 2] : [HD_CollisionHitFireIntern == 2]
    (junction 866) -> CrashFusionAndDetection_SchneeV2_softHit3.Crash [commented out] : %crash scenario 42
        | {
        | CF_scenario = int16(42);
        | }
    (junction 867) -> CrashFusionAndDetection_SchneeV2_softHit3.Crash : %crash scenario 41
        | {
        | CF_scenario = int16(41);
        | }
    (junction 868) -> (junction 873) : %no crash
    (junction 869) -> CrashFusionAndDetection_SchneeV2_softHit3.Crash [order 2] : [RD_fireIntern == 1 && ...
        |  TO_fireIntern == 3]
        | {
        | CF_scenario = int16(32);
        | }
    (junction 871) -> (junction 870)
    (junction 872) -> (junction 871)
    (junction 873) -> (junction 872)
    (junction 874) -> (junction 873)
    (junction 875) -> (junction 874)
    (junction 878) -> CrashFusionAndDetection_SchneeV2_softHit3.Crash : %crash scenario 40
        | {
        | CF_scenario = int16(40);
        | }
    (junction 879) -> CrashFusionAndDetection_SchneeV2_softHit3.Crash : %crash scenario 44
        | {
        | CF_scenario = int16(44);
        | }
    (junction 880) -> CrashFusionAndDetection_SchneeV2_softHit3.Crash : %crash scenario 45
        | {
        | CF_scenario = int16(45);
        | }
    (junction 883) -> CrashFusionAndDetection_SchneeV2_softHit3.Crash : {
        | CF_scenario = int16(80);
        | }
    (junction 884) -> CrashFusionAndDetection_SchneeV2_softHit3.Crash : {
        | CF_scenario = int16(81);
        | }
    (junction 1011) -> CrashFusionAndDetection_SchneeV2_softHit3.Crash : {
        | CF_scenario = int16(82);
        | }
    (junction 1052) -> CrashFusionAndDetection_SchneeV2_softHit3.Crash : {
        | CF_scenario = int16(83);
        | }
    (junction 1015) -> CrashFusionAndDetection_SchneeV2_softHit3.Crash : {
        | CF_scenario = int16(84);
        | }
    (junction 1013) -> CrashFusionAndDetection_SchneeV2_softHit3.Crash : {
        | CF_scenario = int16(85);
        | }
    (junction 1042) -> CrashFusionAndDetection_SchneeV2_softHit3.Crash : {
        | CF_scenario = int16(90);
        | }
    (junction 1043) -> CrashFusionAndDetection_SchneeV2_softHit3.Crash : {
        | CF_scenario = int16(91);
        | }
    (junction 1034) -> CrashFusionAndDetection_SchneeV2_softHit3.Crash : {
        | CF_scenario = int16(92);
        | }
    (junction 1059) -> CrashFusionAndDetection_SchneeV2_softHit3.Crash : {
        | CF_scenario = int16(93);
        | }
    (junction 1031) -> CrashFusionAndDetection_SchneeV2_softHit3.Crash : {
        | CF_scenario = int16(94);
        | }
    (junction 1029) -> CrashFusionAndDetection_SchneeV2_softHit3.Crash : {
        | CF_scenario = int16(95);
        | }
  data: TO_fire input; RD_fire input; CF_fire output; HD_CollisionHitFire input; HD_GroundHitFire input; HD_secondCalibrationDone input; CF_scenario output; CF_checkTipOverTimeDelay local; HD_GroundHitFireIntern local; RRO_fire input; CF_systemConfig input; CF_hubConnection input; RD_fireIntern output; CF_possibleTo output; CF_sdoFire input; TO_fireIntern local; CF_cobiHubSetup input; HD_CollisionHitFireIntern output; CF_bikeStillUpright input
